simulink model "pendulum"  (R2016a)
settings: Solver=VariableStepAuto  StartTime=0.0  StopTime=10.0  RelTol=1e-3
settings Model: Creator=alexalcocer  LastModifiedBy=alexalcocer

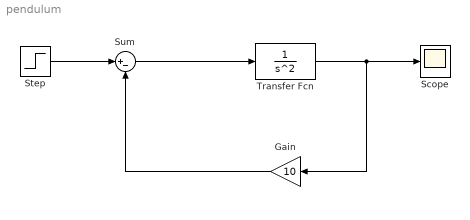
== system pendulum ==
  Gain : Gain  Gain=10
  Scope : Scope
  Step : Step  After=0.01  SampleTime=0
  Sum : Sum  Inputs=|+-
  Transfer Fcn : TransferFcn  Denominator=[1 0 0 ]
  wires:
  Sum/1 -> Transfer Fcn/1
  Gain/1 -> Sum/2
  Transfer Fcn/1 -> Gain/1, Scope/1
  Step/1 -> Sum/1
